simulink model "simulador2017bIDENTIFICATION"  (R2017b)
settings: Solver=FixedStepAuto  StartTime=0.0  StopTime=240  FixedStep=0.01  RelTol=1e-3
values from neighbouring files (symbols this model uses):
  b = 2.9    [FUN.m]    (also in LINEAR_IDENTIFICATION.m = (ThetaX*5+ThetaZ*2)\((accX*5+accZ*2).*mass./S); ratesDerivatives.m = (1/windowSize)*ones(1,windowSize))
  c_bar = 0.19    [FUN.m]
  C_prop = 1    [FUN.m]
  CD_deltae = x(4)    [FUN.m]
  CDp = x(1)    [FUN.m]
  CDq = x(3)    [FUN.m]
  CL0 = x(5)    [FUN.m]
  CL_alpha = x(6)    [FUN.m]
  Cl_beta = x(14)    [FUN.m]
  Cl_da = x(18)    [FUN.m]
  CL_deltae = x(8)    [FUN.m]
  Cl_dr = x(17)    [FUN.m]
  Cl_p = x(15)    [FUN.m]
  Cl_r = x(16)    [FUN.m]
  CLq = x(7)    [FUN.m]
  Cm0 = x(19)    [FUN.m]
  Cm_alpha = x(20)    [FUN.m]
  Cm_de = x(22)    [FUN.m]
  Cm_q = x(21)    [FUN.m]
  Cn_beta = x(23)    [FUN.m]
  Cn_da = x(27)    [FUN.m]
  Cn_dr = x(26)    [FUN.m]
  Cn_p = x(24)    [FUN.m]
  Cn_r = x(25)    [FUN.m]
  Cy_beta = x(9)    [FUN.m]
  Cy_da = x(12)    [FUN.m]
  Cy_dr = x(13)    [FUN.m]
  Cy_p = x(10)    [FUN.m]
  Cy_r = x(11)    [FUN.m]
  k_motor = 80    [FUN.m]
  mass = 11    [FUN.m]
  q = XDATA(:,5)    [FUN.m]    (also in NONLINEAR_IDENTIFICATION.m = myResize(q); fullStateData.mat = [0 -0.00101699788824 -0.00374016767532 -0.00785355630101 -0.; ratesDerivatives.m = q_filt)
  r = XDATA(:,6)    [FUN.m]    (also in NONLINEAR_IDENTIFICATION.m = myResize(r); fullStateData.mat = [-0.0277 -0.0519668037295 -0.0742410523974 -0.0945148626346 ; ratesDerivatives.m = r_filt)
  S = 0.55    [FUN.m]
  Sprop = 0.2027    [FUN.m]
  T = table(xfit,xreal,'RowNames',coeffName)    [NONLINEAR_IDENTIFICATION.m]
undefined symbols (not defined in the file or in its folder): Cl0, Cm_df, Cn0, Cx_df, Cx_dr, Cy0, Cz_df, delta_max, Earth, F, i0, k1, k2, KQ, Kv, Light, M, maxRPM, MIL, N, R, V, Vmax, Vw_unif, WGS84
libraries: aerolibwind2 x3, aerolibtransform2 x2, aerolibasang x2, aerolibfltsims x1, simulink_extras x1, aerolibatmos2 x1, shared6dof x1, aerolibadyn x1
(part 2 of 2)

== system simulador2017bIDENTIFICATION/UAV/Platform /Aircraft Mechanics/Forces & Moments Calculation/Aerodynamic Coefficients /Actuator Increments ==
  Actuator Deflections : Inport  Unit=rad
  deltaeCoef : Inport  Port=2
  Aileron : Subsystem
      mask Display:
      | port_label('input',1,'\delta_a','texmode','on')
      | port_label('output',1,'Y,l,n Coef','texmode','on')
  Elevator : Subsystem
      mask Display:
      | port_label('input',1,'[C_{X_{\delta_e}}, C_{Z_{\delta_e}}]','texmode','on')
      | port_label('input',2,'\delta_e','texmode','on')
      | port_label('output',1,'X, Z, m Coef','texmode','on')
  Flap : Subsystem
      mask Display:
      | port_label('input',1,'\delta_f','texmode','on')
      | port_label('output',1,'X, Z, m Coef','texmode','on')
  Rudder : Subsystem
      mask Display:
      | port_label('input',1,'\delta_r','texmode','on')
      | port_label('output',1,'X,Y,l,n Coef','texmode','on')
  Selector : Selector  InputPortWidth=4  IndexOptions=Index vector (dialog)  Indices=1  OutputSizes=1
  Selector1 : Selector  InputPortWidth=4  IndexOptions=Index vector (dialog)  Indices=2  OutputSizes=1
  Selector2 : Selector  InputPortWidth=4  IndexOptions=Index vector (dialog)  Indices=3  OutputSizes=1
  Selector3 : Selector  InputPortWidth=4  IndexOptions=Index vector (dialog)  Indices=4  OutputSizes=1
  Sum : Sum  Inputs=++++  SaturateOnIntegerOverflow=on  InputSameDT=on  OutDataTypeStr=Inherit: Same as first input
  Coefficients : Outport
  wires:
  Actuator Deflections/1 -> Selector/1, Selector1/1, Selector3/1, Selector2/1
  Aileron/1(delCoeff) -> Sum/1
  Elevator/1(delCoeff) -> Sum/2
  Rudder/1(delCoeff) -> Sum/3
  Flap/1(delCoeff) -> Sum/4
  Sum/1 -> Coefficients/1
  deltaeCoef/1 -> Elevator/1("Cx_deltae, Cz_deltae")
  Selector/1 -> Aileron/1(deltaa)
  Selector1/1 -> Elevator/2(deltae)
  Selector2/1 -> Rudder/1(deltar)
  Selector3/1 -> Flap/1(deltaf)

== system simulador2017bIDENTIFICATION/UAV/Platform /Aircraft Mechanics/Forces & Moments Calculation/Aerodynamic Coefficients /Aerodynamic Actuators ==
  CTRL BUS : Inport
  Bus Selector3 : BusSelector  OutputSignals=deltaa,deltae,deltar,deltaf
  Mux : Mux
  Surface Signals : Outport
  wires:
  Mux/1 -> Surface Signals/1
  Bus Selector3/4 -> Mux/4  "<deltaf>"
  CTRL BUS/1 -> Bus Selector3/1
  Bus Selector3/3 -> Mux/3  "<deltar>"
  Bus Selector3/2 -> Mux/2  "<deltae>"
  Bus Selector3/1 -> Mux/1  "<deltaa>"

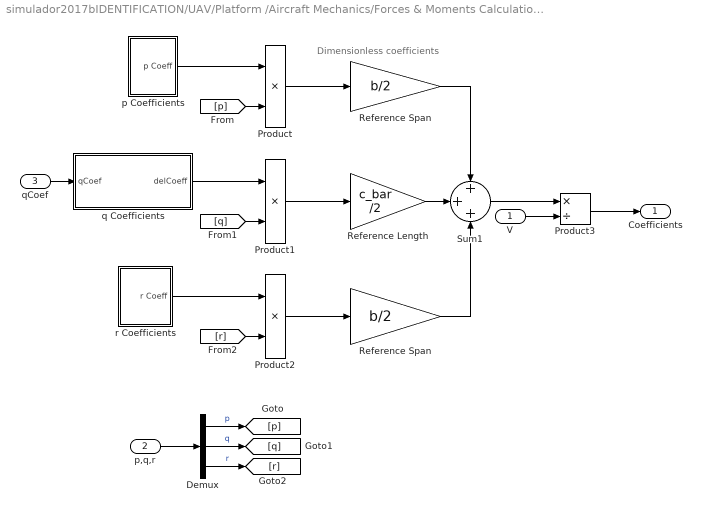
== system simulador2017bIDENTIFICATION/UAV/Platform /Aircraft Mechanics/Forces & Moments Calculation/Aerodynamic Coefficients /Body Rate Damping ==
  note: Dimensionless coefficients
  V : Inport  Unit=m/second
  p,q,r : Inport  Port=2  Unit=rad/second
  "qCoef " : Inport  Port=3
  Demux : Demux  Outputs=3
  Product : Product  SaturateOnIntegerOverflow=on  InputSameDT=on  OutDataTypeStr=Inherit: Same as first input
  Product1 : Product  SaturateOnIntegerOverflow=on  InputSameDT=on  OutDataTypeStr=Inherit: Same as first input
  Product2 : Product  SaturateOnIntegerOverflow=on  InputSameDT=on  OutDataTypeStr=Inherit: Same as first input
  Product3 : Product  Inputs=*/  SaturateOnIntegerOverflow=on  InputSameDT=on  OutDataTypeStr=Inherit: Same as first input
  Reference Length : Gain  Gain=c_bar /2  SaturateOnIntegerOverflow=on  OutDataTypeStr=Inherit: Same as input  ParamDataTypeStr=Inherit: Same as input
  Reference Span : Gain  Gain=b/2  SaturateOnIntegerOverflow=on  OutDataTypeStr=Inherit: Same as input  ParamDataTypeStr=Inherit: Same as input
  "Reference Span " : Gain  Gain=b/2  SaturateOnIntegerOverflow=on  OutDataTypeStr=Inherit: Same as input  ParamDataTypeStr=Inherit: Same as input
  Sum1 : Sum  Inputs=+++  SaturateOnIntegerOverflow=on  InputSameDT=on  OutDataTypeStr=Inherit: Same as first input
  p Coefficients : Subsystem
  q Coefficients : Subsystem
      mask Display:
      | port_label('input',1,'[C_{X_q},C_{Z_q}]','texmode','on')
      | port_label('output',1,'q Coefficients','texmode','on')
  r Coefficients : Subsystem
  Coefficients : Outport
  wires:
  p Coefficients/1(p Coeff) -> Product/1
  q Coefficients/1(delCoeff) -> Product1/1
  p,q,r/1 -> Demux/1
  Demux/1 -> [p]  "p"
  Demux/2 -> [q]  "q"
  Demux/3 -> [r]  "r"
  Sum1/1 -> Product3/1
  V/1 -> Product3/2
  Product3/1 -> Coefficients/1
  Product1/1 -> Reference Length/1
  Product2/1 -> "Reference Span "/1
  Product/1 -> Reference Span/1
  r Coefficients/1(r Coeff) -> Product2/1
  Reference Length/1 -> Sum1/2
  Reference Span/1 -> Sum1/1
  "Reference Span "/1 -> Sum1/3
  "qCoef "/1 -> q Coefficients/1(qCoef)
  [p] -> Product/2
  [q] -> Product1/2
  [r] -> Product2/2

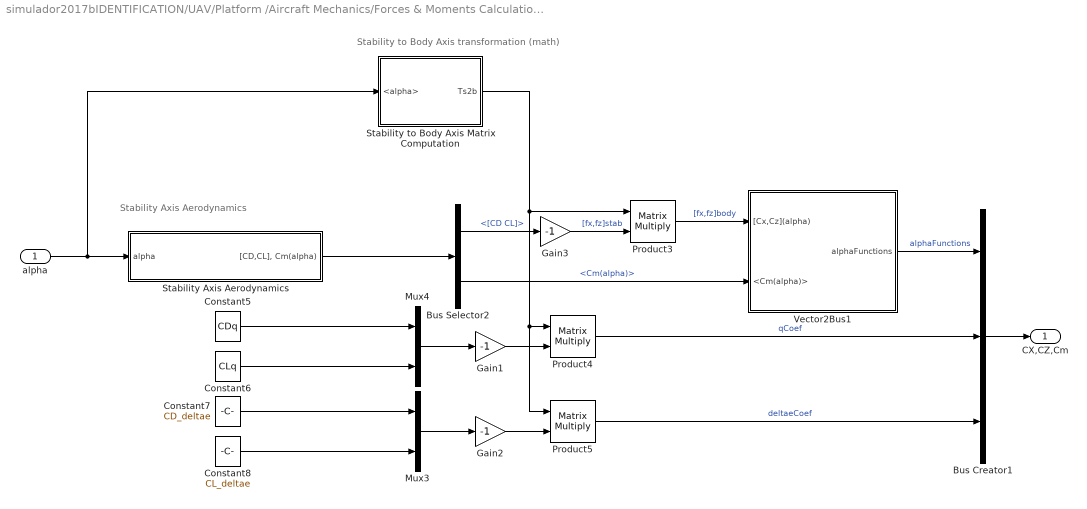
== system simulador2017bIDENTIFICATION/UAV/Platform /Aircraft Mechanics/Forces & Moments Calculation/Aerodynamic Coefficients /Longitudinal Aerodynamics (Cx, Cz, Cm coefficients) ==
  note: Stability Axis Aerodynamics
  note: Stability to Body Axis transformation (math)
  "alpha " : Inport
  Bus Creator1 : BusCreator  Inputs=3
  Bus Selector2 : BusSelector  OutputSignals=[CD CL],Cm(alpha)
  Constant5 : Constant  Value=CDq
      mask Display: port_label('output',1,'C_{D_q}','texmode','on')
  Constant6 : Constant  Value=CLq
      mask Display: port_label('output',1,'C_{L_q}','texmode','on')
  Constant7 : Constant  Value=CD_deltae
      mask Display: port_label('output',1,'C_{D_{\delta_e}}','texmode','on')
  Constant8 : Constant  Value=CL_deltae
      mask Display: port_label('output',1,'C_{L_{\delta_e}}','texmode','on')
  Gain1 : Gain  Gain=-1
  Gain2 : Gain  Gain=-1
  Gain3 : Gain  Gain=-1
  Mux3 : Mux  Inputs=2
  Mux4 : Mux  Inputs=2
  Product3 : Product  Multiplication=Matrix(*)
  Product4 : Product  Multiplication=Matrix(*)
  Product5 : Product  Multiplication=Matrix(*)
  Stability Axis Aerodynamics : Subsystem
      mask Display:
      | port_label('input',1,'\alpha','texmode','on')
      | port_label('output',1,'[C_D(\alpha),C_L(\alpha)], C_m(\alpha)','texmode','on')
  Stability to Body Axis Matrix Computation : Subsystem
      mask Display:
      | port_label('input',1,'\alpha','texmode','on')
      | port_label('output',1,'T_{s2b}(\alpha)','texmode','on')
  Vector2Bus1 : Subsystem
      mask Display:
      | port_label('input',1,'[C_X(\alpha), C_Z(\alpha)]','texmode','on')
      | port_label('input',2,'C_m(\alpha)','texmode','on')
      | port_label('output',1,'C_X(\alpha),C_Z(\alpha),C_m(\alpha)','texmode','on')
  CX,CZ,Cm : Outport
  wires:
  Bus Creator1/1 -> CX,CZ,Cm/1
  Gain3/1 -> Product3/2  "[fx,fz]stab"
  Stability Axis Aerodynamics/1("[CD,CL], Cm(alpha)") -> Bus Selector2/1
  Constant7/1 -> Mux3/1
  Stability to Body Axis Matrix Computation/1(Ts2b) -> Product5/1, Product4/1, Product3/1
  Product4/1 -> Bus Creator1/2  "qCoef"
  Bus Selector2/1 -> Gain3/1  "<[CD CL]>"
  Product5/1 -> Bus Creator1/3  "deltaeCoef"
  Product3/1 -> Vector2Bus1/1("[Cx,Cz](alpha)")  "[fx,fz]body"
  Bus Selector2/2 -> Vector2Bus1/2(<Cm(alpha)>)  "<Cm(alpha)>"
  Constant8/1 -> Mux3/2
  Vector2Bus1/1(alphaFunctions) -> Bus Creator1/1  "alphaFunctions"
  Constant6/1 -> Mux4/2
  Constant5/1 -> Mux4/1
  Mux3/1 -> Gain2/1
  Gain2/1 -> Product5/2
  Mux4/1 -> Gain1/1
  Gain1/1 -> Product4/2
  "alpha "/1 -> Stability Axis Aerodynamics/1(alpha), Stability to Body Axis Matrix Computation/1(<alpha>)

== system simulador2017bIDENTIFICATION/UAV/Platform /Aircraft Mechanics/Forces & Moments Calculation/Aerodynamic Coefficients /alpha-beta Coefficients ==
  beta : Inport  Unit=radian
  Bus Element In : Inport  Port=2  PortName=Longitudinal Aerodynamics  Element=Cm(alpha)
  Bus Element In1 : Inport  Port=2  PortName=Longitudinal Aerodynamics  Element=Cz(alpha)
  Bus Element In2 : Inport  Port=2  PortName=Longitudinal Aerodynamics  Element=Cx(alpha)
  Gain1 : Gain  Gain=Cn_beta  SaturateOnIntegerOverflow=on  OutDataTypeStr=Inherit: Same as input  ParamDataTypeStr=Inherit: Same as input
  Gain3 : Gain  Gain=Cy_beta  SaturateOnIntegerOverflow=on  OutDataTypeStr=Inherit: Same as input  ParamDataTypeStr=Inherit: Same as input
  Gain6 : Gain  Gain=Cl_beta  SaturateOnIntegerOverflow=on  OutDataTypeStr=Inherit: Same as input  ParamDataTypeStr=Inherit: Same as input
  Lateral Dynamics Constants : Constant  Value=[0,Cy0,0,Cl0,0,Cn0]
  Mux1 : Mux  Inputs=6
  Sum4 : Sum  Inputs=|++  SaturateOnIntegerOverflow=on
  Coefficients : Outport
  wires:
  Lateral Dynamics Constants/1 -> Sum4/2
  Sum4/1 -> Coefficients/1
  Mux1/1 -> Sum4/1
  Gain3/1 -> Mux1/2  "Cy"
  Gain6/1 -> Mux1/4  "Cl"
  beta/1 -> Gain1/1, Gain6/1, Gain3/1  "beta"
  Gain1/1 -> Mux1/6
  Bus Element In/1 -> Mux1/5
  Bus Element In1/1 -> Mux1/3
  Bus Element In2/1 -> Mux1/1

== system simulador2017bIDENTIFICATION/UAV/Platform /Aircraft Mechanics/Forces & Moments Calculation/Propulsion/1 dim to 6 dim1 ==
  Tprop : Inport
  Qprop : Inport  Port=2
  Bus Creator : BusCreator  Inputs=2
  Constant : Constant  Value=0
  Mux : Mux  Inputs=3
  Mux1 : Mux  Inputs=3
  Propulsion BUS : Outport
  wires:
  Bus Creator/1 -> Propulsion BUS/1
  Constant/1 -> Mux/3, Mux/2, Mux1/2, Mux1/3
  Qprop/1 -> Mux1/1
  Tprop/1 -> Mux/1
  Mux/1 -> Bus Creator/1  "Tprop"
  Mux1/1 -> Bus Creator/2  "Mprop"

== system simulador2017bIDENTIFICATION/UAV/Platform /Aircraft Mechanics/Forces & Moments Calculation/Propulsion/Motor ==
  Throttle : Inport
  Torque : Inport  Port=2
  Constant : Constant  Value=i0
  Gain : Gain  Gain=Vmax
  Gain1 : Gain  Gain=1/KQ
  Gain2 : Gain  Gain=R/Kv
  Gain3 : Gain  Gain=1/Kv
  Gain4 : Gain  Gain=60/(2*pi)
  Sum : Sum  Inputs=|++
  Sum1 : Sum  Inputs=|+-
  RPM : Outport
  wires:
  Sum/1 -> Gain2/1
  Constant/1 -> Sum/2
  Gain2/1 -> Sum1/2
  Gain/1 -> Gain3/1  "Vin"
  Gain4/1 -> RPM/1  "Omega RPM"
  Throttle/1 -> Gain/1
  Sum1/1 -> Gain4/1  "Omega rad/s"
  Gain3/1 -> Sum1/1
  Gain1/1 -> Sum/1
  Torque/1 -> Gain1/1

== system simulador2017bIDENTIFICATION/UAV/Platform /Aircraft Mechanics/Forces & Moments Calculation/Propulsion/Propeller ==
  RPM : Inport
  u : Inport  Port=2
  1-D Lookup Table : Lookup_n-D  BreakpointsForDimension1=N  BreakpointsForDimension2=V  Table=T+50  InternalRulePriority=Speed  RndMeth=Simplest  InputSameDT=on
  1-D Lookup Table1 : Lookup_n-D  BreakpointsForDimension1=N  BreakpointsForDimension2=V  Table=M  InternalRulePriority=Speed  RndMeth=Simplest  InputSameDT=on
  Tables work with RPM/1000 : Gain  Gain=1/1000
  Tprop : Outport
  Qprop : Outport  Port=2
  wires:
  1-D Lookup Table/1 -> Tprop/1
  u/1 -> 1-D Lookup Table/2, 1-D Lookup Table1/2
  1-D Lookup Table1/1 -> Qprop/1
  RPM/1 -> Tables work with RPM/1000/1
  Tables work with RPM/1000/1 -> 1-D Lookup Table1/1, 1-D Lookup Table/1

== system simulador2017bIDENTIFICATION/UAV/Platform /Aircraft Mechanics/Forces & Moments Calculation/Aerodynamic Coefficients /Actuator Increments/Aileron ==
  note: Se ha despreciado el efecto del angulo de ataque,
      | que afecta a las superficies de control si es muy alto
  deltaa : Inport  Unit=rad
  Gain1 : Gain  Gain=0  SaturateOnIntegerOverflow=on  OutDataTypeStr=Inherit: Same as input  ParamDataTypeStr=Inherit: Same as input
  Gain2 : Gain  Gain=Cy_da  SaturateOnIntegerOverflow=on  OutDataTypeStr=Inherit: Same as input  ParamDataTypeStr=Inherit: Same as input
  Gain3 : Gain  Gain=0  SaturateOnIntegerOverflow=on  OutDataTypeStr=Inherit: Same as input  ParamDataTypeStr=Inherit: Same as input
  Gain4 : Gain  Gain=Cn_da  SaturateOnIntegerOverflow=on  OutDataTypeStr=Inherit: Same as input  ParamDataTypeStr=Inherit: Same as input
  Gain5 : Gain  Gain=0  SaturateOnIntegerOverflow=on  OutDataTypeStr=Inherit: Same as input  ParamDataTypeStr=Inherit: Same as input
  Gain6 : Gain  Gain=Cl_da  SaturateOnIntegerOverflow=on  OutDataTypeStr=Inherit: Same as input  ParamDataTypeStr=Inherit: Same as input
  Mux1 : Mux  Inputs=6
  delCoeff : Outport
  wires:
  Gain6/1 -> Mux1/4
  Gain1/1 -> Mux1/1  "Cx"
  Mux1/1 -> delCoeff/1
  Gain2/1 -> Mux1/2  "Cy"
  Gain3/1 -> Mux1/3  "Cz"
  Gain5/1 -> Mux1/5  "Cm"
  Gain4/1 -> Mux1/6
  deltaa/1 -> Gain2/1, Gain3/1, Gain5/1, Gain4/1, Gain6/1, Gain1/1

== system simulador2017bIDENTIFICATION/UAV/Platform /Aircraft Mechanics/Forces & Moments Calculation/Aerodynamic Coefficients /Actuator Increments/Elevator ==
  "Cx_deltae, Cz_deltae" : Inport
  deltae : Inport  Port=2
  Constant1 : Constant  Value=0
  Demux : Demux  Outputs=2
  Gain3 : Gain  Gain=Cm_de  SaturateOnIntegerOverflow=on  OutDataTypeStr=Inherit: Same as input  ParamDataTypeStr=Inherit: Same as input
  Mux1 : Mux  Inputs=6
  Product : Product
  Product1 : Product
  delCoeff : Outport
  wires:
  Gain3/1 -> Mux1/5
  Product1/1 -> Mux1/3
  Mux1/1 -> delCoeff/1
  Constant1/1 -> Mux1/4, Mux1/6, Mux1/2
  Product/1 -> Mux1/1
  "Cx_deltae, Cz_deltae"/1 -> Demux/1
  Demux/1 -> Product/1  "Cx_deltae"
  Demux/2 -> Product1/1  "Cz_deltae"
  deltae/1 -> Product/2, Product1/2, Gain3/1

== system simulador2017bIDENTIFICATION/UAV/Platform /Aircraft Mechanics/Forces & Moments Calculation/Aerodynamic Coefficients /Actuator Increments/Flap ==
  deltaf : Inport  Unit=rad
  Constant1 : Constant  Value=0
  Gain1 : Gain  Gain=Cx_df  SaturateOnIntegerOverflow=on  OutDataTypeStr=Inherit: Same as input  ParamDataTypeStr=Inherit: Same as input
  Gain3 : Gain  Gain=Cz_df  SaturateOnIntegerOverflow=on  OutDataTypeStr=Inherit: Same as input  ParamDataTypeStr=Inherit: Same as input
  Gain5 : Gain  Gain=Cm_df  SaturateOnIntegerOverflow=on  OutDataTypeStr=Inherit: Same as input  ParamDataTypeStr=Inherit: Same as input
  Mux1 : Mux  Inputs=6
  delCoeff : Outport
  wires:
  deltaf/1 -> Gain1/1, Gain3/1, Gain5/1  "df"
  Gain5/1 -> Mux1/5
  Mux1/1 -> delCoeff/1
  Constant1/1 -> Mux1/4, Mux1/6, Mux1/2
  Gain1/1 -> Mux1/1
  Gain3/1 -> Mux1/3

== system simulador2017bIDENTIFICATION/UAV/Platform /Aircraft Mechanics/Forces & Moments Calculation/Aerodynamic Coefficients /Actuator Increments/Rudder ==
  note: Se añade la contribucion en
      | resistencia del Rudder direccion X
  note: Se ha despreciado el efecto del angulo de ataque,
      | que afecta a las superficies de control si es muy alto
  deltar : Inport  Unit=rad
  Constant1 : Constant  Value=0
  Gain1 : Gain  Gain=Cl_dr  SaturateOnIntegerOverflow=on  OutDataTypeStr=Inherit: Same as input  ParamDataTypeStr=Inherit: Same as input
  Gain2 : Gain  Gain=Cn_dr  SaturateOnIntegerOverflow=on  OutDataTypeStr=Inherit: Same as input  ParamDataTypeStr=Inherit: Same as input
  Gain4 : Gain  Gain=Cy_dr  SaturateOnIntegerOverflow=on  OutDataTypeStr=Inherit: Same as input  ParamDataTypeStr=Inherit: Same as input
  Gain5 : Gain  Commented=on  Gain=Cx_dr  SaturateOnIntegerOverflow=on  OutDataTypeStr=Inherit: Same as input  ParamDataTypeStr=Inherit: Same as input
  Mux1 : Mux  Inputs=6
  delCoeff : Outport
  wires:
  Gain1/1 -> Mux1/4
  Gain2/1 -> Mux1/6
  Mux1/1 -> delCoeff/1
  Gain4/1 -> Mux1/2
  Constant1/1 -> Mux1/1, Mux1/5, Mux1/3
  deltar/1 -> Gain5/1, Gain4/1, Gain1/1, Gain2/1  "dr"

== system simulador2017bIDENTIFICATION/UAV/Platform /Aircraft Mechanics/Forces & Moments Calculation/Aerodynamic Coefficients /Body Rate Damping/p Coefficients ==
  Constant1 : Constant  Value=0
  Constant2 : Constant  Value=Cy_p
  Constant3 : Constant  Value=Cl_p
  Constant4 : Constant  Value=Cn_p
  Mux1 : Mux  Inputs=6
  p Coeff : Outport
  wires:
  Constant2/1 -> Mux1/2
  Mux1/1 -> p Coeff/1
  Constant1/1 -> Mux1/5, Mux1/3, Mux1/1
  Constant4/1 -> Mux1/6
  Constant3/1 -> Mux1/4

== system simulador2017bIDENTIFICATION/UAV/Platform /Aircraft Mechanics/Forces & Moments Calculation/Aerodynamic Coefficients /Body Rate Damping/q Coefficients ==
  qCoef : Inport
  Constant1 : Constant  Value=0
  Constant4 : Constant  Value=Cm_q
  Demux : Demux  Outputs=2
  Mux1 : Mux  Inputs=6
  delCoeff : Outport
  wires:
  Constant1/1 -> Mux1/6, Mux1/4, Mux1/2
  Constant4/1 -> Mux1/5
  Mux1/1 -> delCoeff/1
  qCoef/1 -> Demux/1
  Demux/1 -> Mux1/1  "Cx_q"
  Demux/2 -> Mux1/3  "Cz_q"

== system simulador2017bIDENTIFICATION/UAV/Platform /Aircraft Mechanics/Forces & Moments Calculation/Aerodynamic Coefficients /Body Rate Damping/r Coefficients ==
  Constant : Constant  Value=0
  Constant1 : Constant  Value=Cy_r
  Constant2 : Constant  Value=Cl_r
  Constant4 : Constant  Value=Cn_r
  Mux1 : Mux  Inputs=6
  r Coeff : Outport
  wires:
  Constant/1 -> Mux1/5, Mux1/3, Mux1/1
  Constant1/1 -> Mux1/2
  Constant4/1 -> Mux1/6
  Constant2/1 -> Mux1/4
  Mux1/1 -> r Coeff/1

== system simulador2017bIDENTIFICATION/UAV/Platform /Aircraft Mechanics/Forces & Moments Calculation/Aerodynamic Coefficients /Longitudinal Aerodynamics (Cx, Cz, Cm coefficients)/Stability Axis Aerodynamics ==
  note: CD
  alpha : Inport
  Constant1 : Constant  Value=CL0
  Constant2 : Constant  Value=Cm0
  Constant3 : Constant  Value=CDp
  Gain1 : Gain  Gain=k1
  Gain2 : Gain  Gain=k2
  Gain4 : Gain  Gain=CL_alpha
  Gain5 : Gain  Gain=Cm_alpha
  Math Function : Math  Operator=square  SaturateOnIntegerOverflow=on
  Mux : Mux  Inputs=3
  Sum : Sum  Inputs=|++
  Sum1 : Sum  Inputs=|++
  Sum2 : Sum  Inputs=+++
  Vector2Bus : Subsystem
  "[CD,CL], Cm(alpha)" : Outport
  wires:
  Gain4/1 -> Sum/1
  Gain5/1 -> Sum1/1
  Vector2Bus/1("[CD,CL], Cm") -> "[CD,CL], Cm(alpha)"/1
  Constant1/1 -> Sum/2
  Constant2/1 -> Sum1/2
  Sum1/1 -> Mux/3  "Cm"
  Mux/1 -> Vector2Bus/1("[CD,CL,Cm]")
  Sum2/1 -> Mux/1  "CD"
  Sum/1 -> Gain2/1, Math Function/1, Mux/2  "CL"
  Constant3/1 -> Sum2/3
  alpha/1 -> Gain5/1, Gain4/1
  Gain2/1 -> Sum2/2
  Math Function/1 -> Gain1/1  "CL2"
  Gain1/1 -> Sum2/1

== system simulador2017bIDENTIFICATION/UAV/Platform /Aircraft Mechanics/Forces & Moments Calculation/Aerodynamic Coefficients /Longitudinal Aerodynamics (Cx, Cz, Cm coefficients)/Stability to Body Axis Matrix Computation ==
  note: [ ]
  note: sin cos
  note: cos -sin
  note: Column 2
  note: Column 1
  <alpha> : Inport
  Cos1 : Trigonometry  Operator=cos  OutputSignalType=real
  Cos2 : Trigonometry  OutputSignalType=real
  Gain : Gain  Gain=-1
  Matrix Concatenate : Concatenate  Mode=Multidimensional array  ConcatenateDimension=2
  Mux : Mux  Inputs=2
  Mux3 : Mux  Inputs=2
  Test Display : Display
  Ts2b : Outport
  wires:
  Gain/1 -> Mux/1
  Cos2/1 -> Mux3/2, Gain/1
  Mux3/1 -> Matrix Concatenate/1
  Mux/1 -> Matrix Concatenate/2
  Cos1/1 -> Mux3/1, Mux/2
  <alpha>/1 -> Cos2/1, Cos1/1
  Matrix Concatenate/1 -> Test Display/1, Ts2b/1  "Ts2b"

== system simulador2017bIDENTIFICATION/UAV/Platform /Aircraft Mechanics/Forces & Moments Calculation/Aerodynamic Coefficients /Longitudinal Aerodynamics (Cx, Cz, Cm coefficients)/Vector2Bus1 ==
  "[Cx,Cz](alpha)" : Inport
  <Cm(alpha)> : Inport  Port=2
  Bus Creator : BusCreator  Inputs=3
  Demux : Demux  Outputs=2
  alphaFunctions : Outport
  wires:
  "[Cx,Cz](alpha)"/1 -> Demux/1
  <Cm(alpha)>/1 -> Bus Creator/3
  Demux/2 -> Bus Creator/2  "Cz(alpha)"
  Demux/1 -> Bus Creator/1  "Cx(alpha)"
  Bus Creator/1 -> alphaFunctions/1  "alphaFunctions"

== system simulador2017bIDENTIFICATION/UAV/Platform /Aircraft Mechanics/Forces & Moments Calculation/Aerodynamic Coefficients /Longitudinal Aerodynamics (Cx, Cz, Cm coefficients)/Stability Axis Aerodynamics/Vector2Bus ==
  "[CD,CL,Cm]" : Inport
  Bus Creator : BusCreator  Inputs=2
  Demux : Demux  Outputs=3
  Mux1 : Mux  Inputs=2
  "[CD,CL], Cm" : Outport
  wires:
  Demux/3 -> Bus Creator/2  "Cm(alpha)"
  Demux/1 -> Mux1/1  "CD"
  Mux1/1 -> Bus Creator/1  "[CD CL]"
  "[CD,CL,Cm]"/1 -> Demux/1
  Bus Creator/1 -> "[CD,CL], Cm"/1
  Demux/2 -> Mux1/2  "CL"

== matlab function simulador2017bIDENTIFICATION/UAV/Flight Data Recorder (FDR)/IMU Sensor Recorder/Accelerometer + Noise ==
  settings: updateMethod=DISCRETE  sampleTime=0.01
  data: rho input; accX output; Va input; deltat input; Cx input; Cy input; Cz input; accY output; accZ output; S parameter; mass parameter; Sprop parameter; C_prop parameter; k_motor parameter
function [accX,accY,accZ] = fcn(rho,Va,deltat,Cx,Cy,Cz,S,mass,Sprop,C_prop,k_motor)
% noise is 25% of the signal amplitude
a0      = rho*Va*Va*S/(2*mass);
aprop   = rho*Sprop*C_prop/(2*mass);
%% X measurement
accX_clean  = a0*Cx + aprop*((k_motor*deltat)^2-Va^2); 
max_X       = 0.02*2; % Maximum acceleration amplitude in X
noiseX      = max_X*0.25*(-1+2*rand(1));

accX        = accX_clean + noiseX;
%% Y measurement
accY_clean  = a0*Cy; 
max_Y       = 1e-3*2; % Maximum acceleration amplitude in Y
noiseY      = max_Y*0.25*(-1+2*rand(1)); 

accY        = accY_clean + noiseY;

%% Z measurement
accZ_clean  = a0*Cz;
max_Z       = 9.8/2; % Maximum acceleration amplitude in Z
noiseZ      = max_Z*0.25*(-1+2*rand(1));

accZ        = accZ_clean + noiseZ;

== matlab function simulador2017bIDENTIFICATION/Scopes/Visualization BOX/Cockpit Data/MATLAB Function ==
  data: uvw input; airspeed output
function airspeed = fcn(uvw)

u = uvw(1);
v = uvw(2);
w = uvw(3);

airspeed = sqrt(u^2+v^2+w^2);
airspeed = airspeed*1.94384449; % unit convertion

== matlab function simulador2017bIDENTIFICATION/UAV/Flight Data Recorder (FDR)/IMU Sensor Recorder/Gyro + Noise ==
  settings: updateMethod=DISCRETE  sampleTime=0.01
  data: p input; p_meas output; q input; r input; q_meas output; r_meas output
function [p_meas,q_meas,r_meas] = fcn(p,q,r)
% rng('default') reset de rand() settings so that they produce the same
% random numbers as if you restarted MATLAB. Doing this 3 times ensures
% that the noise added to each gyro signal is independent of each other.
nu=2.5;
noise      = nu*pi/180*(-1+2*rand(1));
%% X measurement
p_meas      = p + noise;
%% Y measurement
q_meas        = q + noise;
%% Z measurement
r_meas        = r + noise;

== matlab function simulador2017bIDENTIFICATION/UAV/Flight Data Recorder (FDR)/Other Sensors Recorder/Angle Noise ==
  data: y_clean output; u input; y output
function [y_clean,y] = fcn(u)
y_clean = u;
max_u=0.*pi./180;
noise = max_u.*.5.*(-1+2.*rand(1)); % rand num (-1,1)*(50% of u)->(-50%,50%) of u
y = u+ noise;

== matlab function simulador2017bIDENTIFICATION/UAV/Flight Data Recorder (FDR)/Other Sensors Recorder/Va Noise ==
  data: y_clean output; u input; y output
function [y_clean,y] = fcn(u)
y_clean = u;
max_u=0;
noise = max_u.*.2.*(-1+2.*rand(1)); % rand num (-1,1)*(50% of u)->(-20%,20%) of u
y = u+ noise;

== matlab function simulador2017bIDENTIFICATION/UAV/Flight Data Recorder (FDR)/Other Sensors Recorder/control surfaces ==
  data: y_clean output; u input; y output
function [y_clean,y] = fcn(u)
y_clean = u;
max_u=0*pi/180;
noise = max_u.*.15.*(-1+2.*rand(1)); % rand num (-1,1)*(15% of u)->(-15%,15%) of u
y = u+ noise;

== matlab function simulador2017bIDENTIFICATION/UAV/Flight Data Recorder (FDR)/Other Sensors Recorder/air density ==
  data: y_clean output; u input; y output
function [y_clean,y] = fcn(u)
y_clean = u;
max_u=0;
noise = max_u.*.2.*(-1+2.*rand(1)); % rand num (-1,1)*(20% of u)->(-20%,20%) of u
y = u+ noise;

== matlab function simulador2017bIDENTIFICATION/UAV/Flight Data Recorder (FDR)/Other Sensors Recorder/thrust ==
  data: y_clean output; u input; y output
function [y_clean,y] = fcn(u)
y_clean = u;
max_u=0;
noise = max_u.*.2.*(-1+2.*rand(1)); % rand num (-1,1)*(20% of u)->(-20%,20%) of u
y = u+ noise;
